simulink model "fir_filter"  (R2022b)
settings: Solver=FixedStepAuto  StartTime=0.0  StopTime=10.0  FixedStep=0.001  RelTol=1e-3
libraries: simulink x1
settings Model: Creator=rherz  LastModifiedBy=rherz
settings OptimizationCC: DefaultParameterBehavior=Inlined  EnhancedBackFolding=on  PassReuseOutputArgsAs=Individual arguments  ZeroExternalMemoryAtStartup=off  ZeroInternalMemoryAtStartup=off  OptimizeBlockOrder=speed  DifferentSizesBufferReuse=on  EfficientTunableParamExpr=on
settings DebuggingCC: ParameterTunabilityLossMsg=error
settings HardwareCC: ProdBitPerPointer=32  ProdBitPerSizeT=32  ProdBitPerPtrDiffT=32  ProdLargestAtomicInteger=Long  ProdLargestAtomicFloat=Double  ProdWordSize=32  ProdHWDeviceType=ARM Compatible->ARM Cortex-A
settings SFSimCC: MATLABDynamicMemAlloc=off
settings RTWCC: Description=Embedded Coder  SystemTargetFile=ert.tlc  GenCodeOnly=on  TemplateMakefile=ert_default_tmf
settings CodeAppCC: ForceParamTrailComments=on  IgnoreCustomStorageClasses=off  OperatorAnnotations=on  SimulinkDataObjDesc=on  SFDataObjDesc=on  InsertBlockDesc=on
settings ERTTargetCC: TargetLangStandard=C99 (ISO)  GenerateSampleERTMain=on  InlinedParameterPlacement=NonHierarchical  ERTCustomFileTemplate=example_file_process.tlc

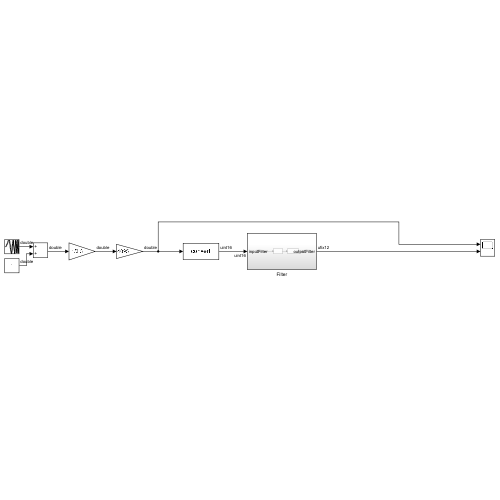
[thumbnail: Simulink's stored preview of the top-level diagram]
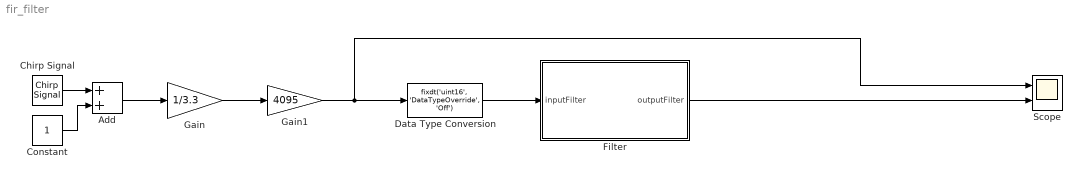
== system fir_filter ==
  Add : Sum
  Chirp Signal : simulink/Sources/Chirp Signal  f1=0  T=10  f2=1000
  Constant : Constant
  Data Type Conversion : DataTypeConversion  OutDataTypeStr=fixdt('uint16', 'DataTypeOverride', 'Off')  RndMeth=Floor
  Filter : Subsystem
  Gain : Gain  Gain=1/3.3
  Gain1 : Gain  Gain=4095
  Scope : Scope  NumInputPorts=2
  wires:
  Chirp Signal/1 -> Add/1
  Constant/1 -> Add/2
  Add/1 -> Gain/1
  Gain/1 -> Gain1/1
  Data Type Conversion/1 -> Filter/1(inputFilter)
  Filter/1(outputFilter) -> Scope/2
  Gain1/1 -> Scope/1, Data Type Conversion/1

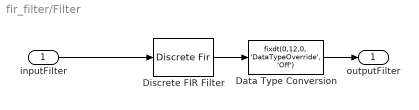
== system fir_filter/Filter ==
  inputFilter : Inport  OutDataTypeStr=fixdt('uint16', 'DataTypeOverride', 'Off')
  Data Type Conversion : DataTypeConversion  OutDataTypeStr=fixdt(0,12,0, 'DataTypeOverride', 'Off')  RndMeth=Floor
  Discrete FIR Filter : DiscreteFir  Coefficients=[-0.022941089669897156 -0.041759395677959277 -0.047725023631953453 -0.034411634504845724 0.000000000000000009 0.051617451757268590 0.111358388474558048 0.167037582711837107 0.206469807029074304 0.220707827023835096 0.206469807029074304 0.167037582711837107 0.111358388474558048 0.051617451757268590 0.000000000000000009 -0.034411634504845724 -0.047725023631953453 -0.041759395677959277 -0.022941089669897156]  SampleTime=0.001  CoefDataTypeStr=fixdt(1,32,30, 'DataTypeOverride', 'Off')  ProductDataTypeStr=fixdt(1,32,10, 'DataTypeOverride', 'Off')  AccumDataTypeStr=fixdt(1,32,10, 'DataTypeOverride', 'Off')  OutDataTypeStr=fixdt('int32', 'DataTypeOverride', 'Off')
  outputFilter : Outport
  wires:
  inputFilter/1 -> Discrete FIR Filter/1
  Discrete FIR Filter/1 -> Data Type Conversion/1
  Data Type Conversion/1 -> outputFilter/1
